simulink model "sogi_validation"  (R2026a)
settings: Solver=ode45  StopTime=1  MaxStep=double(Cal_SOGI_Ts_s_f32)/8  RelTol=1e-9  AbsTol=1e-11
PostLoadFcn:
  | addpath(fileparts(get_param('sogi_validation','FileName'))); sogi_refresh_parameter_panels('sogi_validation');
InitFcn:
  | sogi_check_parameter_binding('sogi_validation',false);
StartFcn:
  | sogi_check_parameter_binding('sogi_validation',true,true);
values from neighbouring files (symbols this model uses):
  Cal_SOGI_F0_Hz_f32 = 50.0    [sogi_parameters.sldd]
  Cal_SOGI_K_f32 = 1.41421354    [sogi_parameters.sldd]
  Cal_SOGI_Ts_s_f32 = 5.0E-5    [sogi_parameters.sldd]
settings Model: DataDictionary=sogi_parameters.sldd  EnableAccessToBaseWorkspace=off  Creator=ASUS  LastModifiedBy=ASUS

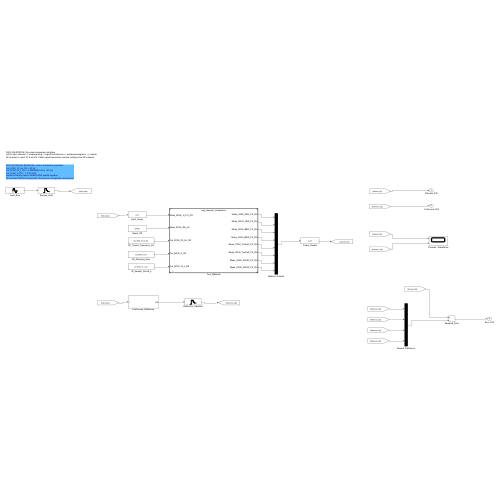
[thumbnail: Simulink's stored preview of the top-level diagram]
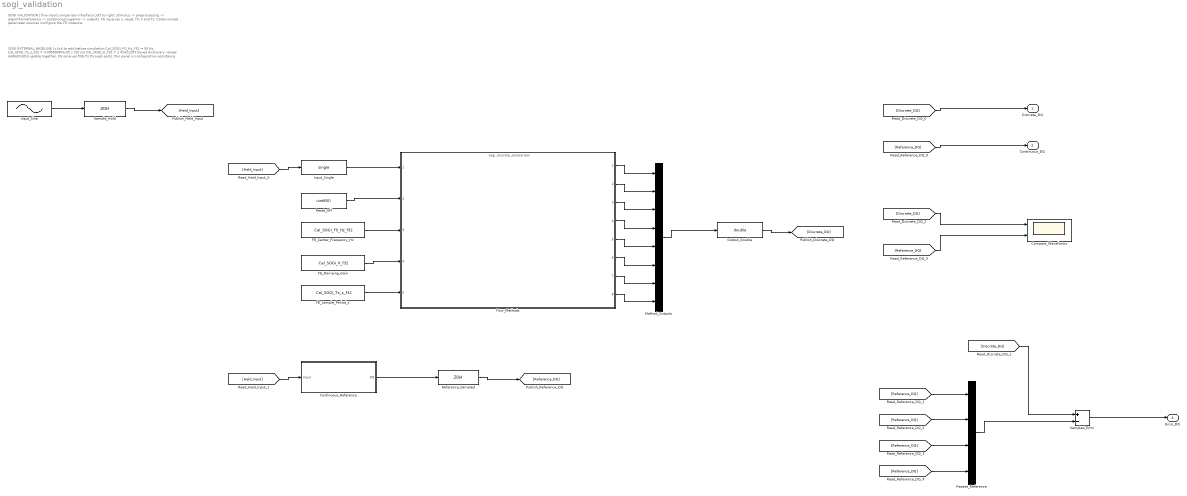
== system sogi_validation ==
  note: SOGI VALIDATION | five-input comparison interface
      | Left to right: stimulus -> preprocessing -> algorithm/reference -> postprocessing/error -> outputs.
      | FE receives u, reset, f0, k and Ts. Caller-owned parameter sources configure the FE instance.
  note: SOGI EXTERNAL BASELINE | click to edit before simulation
      | Cal_SOGI_F0_Hz_f32 = 50 Hz
      | Cal_SOGI_Ts_s_f32 = 4.99999987e-05 s  (50 us)
      | Cal_SOGI_K_f32 = 1.41421354
      | Saved dictionary values; Ad/Bd/Cd/Dd update together.
      | FE receives f0/k/Ts through ports; this panel is configuration assistance.
  Compare_Waveforms : Scope  NumInputPorts=2
      settings: ActiveDisplayYMinimum=-1.1948721553316026  ActiveDisplayYMaximum=-0.53758119877036681
  Continuous_Reference : Subsystem
  FE_Center_Frequency_Hz : Constant  Value=Cal_SOGI_F0_Hz_f32  OutDataTypeStr=single
  FE_Damping_Gain : Constant  Value=Cal_SOGI_K_f32  OutDataTypeStr=single
  FE_Sample_Period_s : Constant  Value=Cal_SOGI_Ts_s_f32  OutDataTypeStr=single
  Four_Methods : ModelReference  ModelNameDialog=sogi_discrete_comparison  SimulationMode=Normal  ModelReferenceVersion=1.21
  Input_Sine : Sin  Frequency=2*pi*double(Cal_SOGI_F0_Hz_f32)  SampleTime=0
  Input_Single : DataTypeConversion  OutDataTypeStr=single  SaturateOnIntegerOverflow=off  RndMeth=Floor
  Method_Outputs : Mux  Inputs=8
  Output_Double : DataTypeConversion  OutDataTypeStr=double  SaturateOnIntegerOverflow=off  RndMeth=Floor
  Reference_Sampled : ZeroOrderHold  SampleTime=double(Cal_SOGI_Ts_s_f32)
  Repeat_Reference : Mux
  Reset_Off : Constant  Value=uint8(0)  OutDataTypeStr=uint8  SampleTime=double(Cal_SOGI_Ts_s_f32)
  Sample_Hold : ZeroOrderHold  SampleTime=double(Cal_SOGI_Ts_s_f32)
  Sampled_Error : Sum  Inputs=+-
  Discrete_DQ : Outport
  Continuous_DQ : Outport  Port=2
  Error_DQ : Outport  Port=3
  wires:
  [Discrete_DQ] -> Compare_Waveforms/1
  [Discrete_DQ] -> Sampled_Error/1
  [Discrete_DQ] -> Discrete_DQ/1
  [Reference_DQ] -> Compare_Waveforms/2
  [Reference_DQ] -> Repeat_Reference/4
  [Reference_DQ] -> Repeat_Reference/3
  [Reference_DQ] -> Repeat_Reference/2
  [Reference_DQ] -> Repeat_Reference/1
  [Reference_DQ] -> Continuous_DQ/1
  [Held_Input] -> Continuous_Reference/1(Input)
  [Held_Input] -> Input_Single/1
  Input_Sine/1 -> Sample_Hold/1
  Sample_Hold/1 -> [Held_Input]
  Input_Single/1 -> Four_Methods/1
  Reset_Off/1 -> Four_Methods/2
  Reference_Sampled/1 -> [Reference_DQ]
  Method_Outputs/1 -> Output_Double/1
  Output_Double/1 -> [Discrete_DQ]
  Repeat_Reference/1 -> Sampled_Error/2
  Sampled_Error/1 -> Error_DQ/1
  Four_Methods/1 -> Method_Outputs/1
  Four_Methods/2 -> Method_Outputs/2
  Four_Methods/3 -> Method_Outputs/3
  Four_Methods/4 -> Method_Outputs/4
  Four_Methods/5 -> Method_Outputs/5
  Four_Methods/6 -> Method_Outputs/6
  Four_Methods/7 -> Method_Outputs/7
  Four_Methods/8 -> Method_Outputs/8
  Continuous_Reference/1(DQ) -> Reference_Sampled/1
  FE_Sample_Period_s/1 -> Four_Methods/5
  FE_Damping_Gain/1 -> Four_Methods/4
  FE_Center_Frequency_Hz/1 -> Four_Methods/3

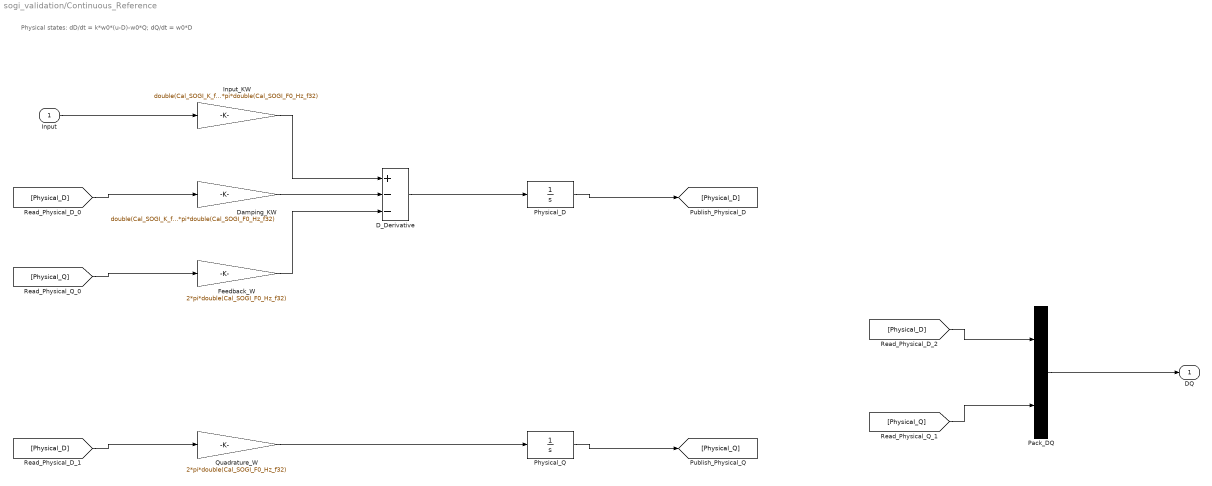
== system sogi_validation/Continuous_Reference ==
  note: Physical states: dD/dt = k*w0*(u-D)-w0*Q; dQ/dt = w0*D
  Input : Inport
  D_Derivative : Sum  Inputs=+--
  Damping_KW : Gain  Gain=double(Cal_SOGI_K_f32)*2*pi*double(Cal_SOGI_F0_Hz_f32)
  Feedback_W : Gain  Gain=2*pi*double(Cal_SOGI_F0_Hz_f32)
  Input_KW : Gain  Gain=double(Cal_SOGI_K_f32)*2*pi*double(Cal_SOGI_F0_Hz_f32)
  Pack_DQ : Mux  Inputs=2
  Physical_D : Integrator
  Physical_Q : Integrator
  Quadrature_W : Gain  Gain=2*pi*double(Cal_SOGI_F0_Hz_f32)
  DQ : Outport
  wires:
  [Physical_Q] -> Pack_DQ/2
  [Physical_Q] -> Feedback_W/1
  [Physical_D] -> Pack_DQ/1
  [Physical_D] -> Quadrature_W/1
  [Physical_D] -> Damping_KW/1
  Quadrature_W/1 -> Physical_Q/1
  D_Derivative/1 -> Physical_D/1
  Feedback_W/1 -> D_Derivative/3
  Physical_Q/1 -> [Physical_Q]
  Damping_KW/1 -> D_Derivative/2
  Physical_D/1 -> [Physical_D]
  Input_KW/1 -> D_Derivative/1
  Input/1 -> Input_KW/1
  Pack_DQ/1 -> DQ/1
